simulink model "TestSupervisorFSM_TX"  (R2024b)
settings: Solver=FixedStepDiscrete  StartTime=0.0  StopTime=inf  FixedStep=0.001  RelTol=1e-3  EnableMultiTasking=on
model workspace (MAT data in the model file):
  Command = 1
  State = 0
undefined symbols (not defined in the file): ControlModes
libraries: eeStairGenerator x6
settings Model: DataDictionary=embeddedBoard_common.sldd  Creator=vvasco  LastModifiedBy=mfussi
settings SolverCC: AlgebraicLoopSolver=TrustRegion  AutoInsertRateTranBlk=on
settings DataIOCC: LimitDataPoints=on
settings OptimizationCC: ReuseModelBlockBuffer=off  LifeSpan=inf
settings DebuggingCC: ParameterPrecisionLossMsg=none  UnconnectedInputMsg=warning  UnconnectedOutputMsg=warning  UnconnectedLineMsg=warning  AllowSymbolicDim=off  SFUnexpectedBacktrackingDiag=warning  SFNoUnconditionalDefaultTransitionDiag=warning  SFExecutionAtInitializationDiag=none  ArithmeticOperatorsInVariantConditions=warning
settings ModelReferenceCC: EnableRefExpFcnMdlSchedulingChecks=on
settings SFSimCC: SimUseLocalCustomCode=off  CustomCodeUndefinedFunction=UseInterfaceOnly
settings RTWCC: RTWUseLocalCustomCode=off  GPUComputeCapability=3.5  DLArmComputeVersion=19.05
settings CodeAppCC: StateflowObjectComments=on
settings GRTTargetCC: TargetLangStandard=C89/C90 (ANSI)
settings ConfigComp: CovMetricSettings=dw  CovSaveCumulativeToWorkspaceVar=on  CovSaveSingleToWorkspaceVar=on  CovExternalEMLEnable=off

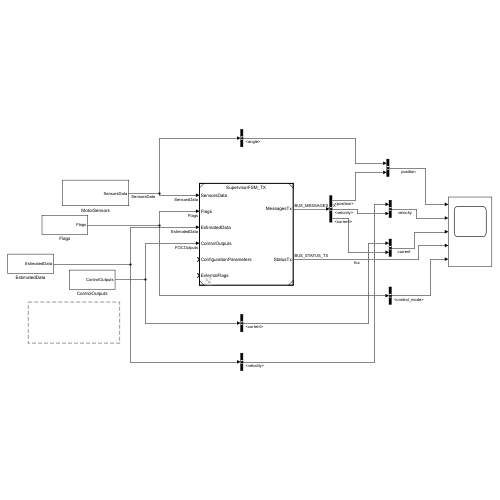
[thumbnail: Simulink's stored preview of the top-level diagram]
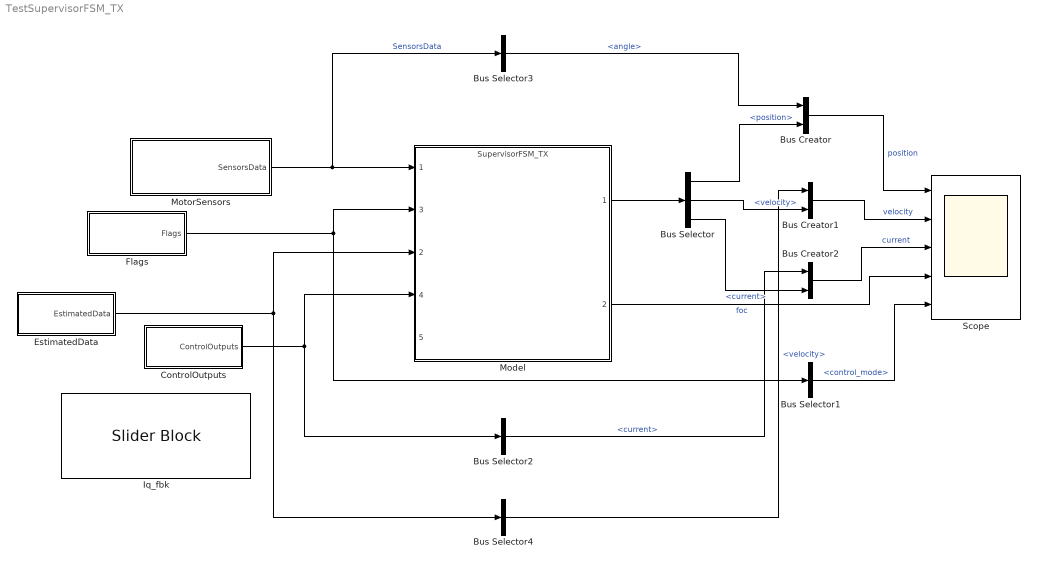
== system TestSupervisorFSM_TX ==
  Bus Creator : BusCreator  Inputs=2
  Bus Creator1 : BusCreator  Inputs=2
  Bus Creator2 : BusCreator  Inputs=2
  Bus Selector : BusSelector  OutputSignals=foc.position,foc.velocity,foc.current
  Bus Selector1 : BusSelector  OutputSignals=control_mode
  Bus Selector2 : BusSelector  OutputSignals=Iq_fbk.current
  Bus Selector3 : BusSelector  OutputSignals=motorsensors.angle
  Bus Selector4 : BusSelector  OutputSignals=jointvelocities.velocity
  ControlOutputs : Subsystem
  EstimatedData : Subsystem
  Flags : Subsystem
  Iq_fbk : SliderBlock  ScaleMax=20
  Model : ModelReference  ModelNameDialog=SupervisorFSM_TX.slx  SimulationMode=Normal  ModelReferenceVersion=9.0
      settings: PortSchema="{\"entries\":[{\"content\":{\"sides\":[{\"content\":{\"connectorIds\":[\"In1\",\"In3\",\"In2\",\"In4\",\"In5\"]},\"type\":\"ConnectorPlacement.EquallySpacedRectSide\",\"uuid\":\"69e4ef43-4003-4440-a894-3828c1af5902\"},{\"content\":{\"connectorIds\":[\"Out1\",\"Out2\"],\"side\":\"RIGHT\"},\"type\":\"ConnectorPlacement.EquallySpacedRectSide\",\"uuid\":\"4c041ecf-670d-4f38-bad4-7d246327a855\"},{\"content\":{\"side\":\"TOP\"},\"type\":\"ConnectorPlacement.EquallySpacedRectSide\",\"uuid\":\"dbbb66c6-d08b-4ab5-92ab-8954eaf6e6e2\"}]},\"type\":\"ConnectorPlacement.EquallySpacedConnector\",\"uuid\":\"4940a0b0-17cd-4df8-8277-6fa028eccbd4\"}],\"packageUris\":[\"http://schema.mathworks.com/mf0/Connector/R2020b\"],\"version\":\"1.0\"}"
  MotorSensors : Subsystem
  Scope : Scope  NumInputPorts=5
  wires:
  Bus Selector/1 -> Bus Creator/2  "<position>"
  Bus Selector3/1 -> Bus Creator/1  "<angle>"
  Bus Creator/1 -> Scope/1  "position"
  Bus Creator1/1 -> Scope/2  "velocity"
  Bus Selector/2 -> Bus Creator1/2  "<velocity>"
  Bus Selector/3 -> Bus Creator2/2  "<current>"
  Bus Creator2/1 -> Scope/3  "current"
  Bus Selector1/1 -> Scope/5  "<control_mode>"
  Model/2 -> Scope/4  "foc"
  Model/1 -> Bus Selector/1
  ControlOutputs/1(ControlOutputs) -> Model/4, Bus Selector2/1
  EstimatedData/1(EstimatedData) -> Model/2, Bus Selector4/1
  MotorSensors/1(SensorsData) -> Bus Selector3/1, Model/1  "SensorsData"
  Bus Selector2/1 -> Bus Creator2/1  "<current>"
  Bus Selector4/1 -> Bus Creator1/1  "<velocity>"
  Flags/1(Flags) -> Bus Selector1/1, Model/3

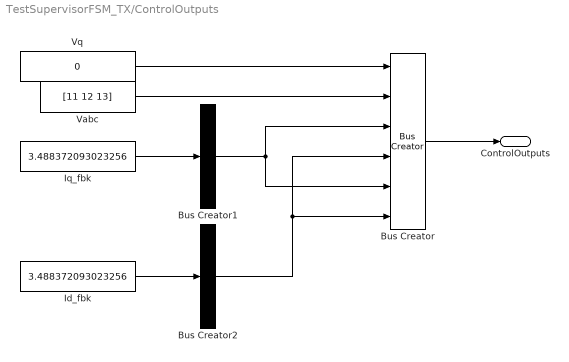
== system TestSupervisorFSM_TX/ControlOutputs ==
  Bus Creator : BusCreator  Inputs=6  OutDataTypeStr=Bus: ControlOutputs
      settings: InheritFromInputs=off
  Bus Creator1 : BusCreator  Inputs=1  OutDataTypeStr=Bus: MotorCurrent
      settings: InheritFromInputs=off
  Bus Creator2 : BusCreator  Inputs=1  OutDataTypeStr=Bus: MotorCurrent
      settings: InheritFromInputs=off
  Id_fbk : Constant  Value=3.488372093023256  OutDataTypeStr=single
  Iq_fbk : Constant  Value=3.488372093023256  OutDataTypeStr=single
  Vabc : Constant  Value=[11 12 13]  OutDataTypeStr=single
  Vq : Constant  Value=0  OutDataTypeStr=single
  ControlOutputs : Outport  OutDataTypeStr=Bus: ControlOutputs
  wires:
  Iq_fbk/1 -> Bus Creator1/1
  Bus Creator/1 -> ControlOutputs/1
  Bus Creator1/1 -> Bus Creator/5, Bus Creator/3
  Vabc/1 -> Bus Creator/2
  Vq/1 -> Bus Creator/1
  Bus Creator2/1 -> Bus Creator/6, Bus Creator/4
  Id_fbk/1 -> Bus Creator2/1

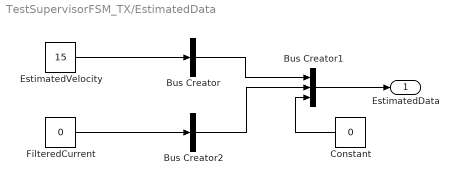
== system TestSupervisorFSM_TX/EstimatedData ==
  Bus Creator : BusCreator  Inputs=1  OutDataTypeStr=Bus: JointVelocities  NonVirtualBus=on
      settings: InheritFromInputs=off
  Bus Creator1 : BusCreator  Inputs=3  OutDataTypeStr=Bus: EstimatedData  NonVirtualBus=on
      settings: InheritFromInputs=off
  Bus Creator2 : BusCreator  Inputs=1  OutDataTypeStr=Bus: MotorCurrent  NonVirtualBus=on
      settings: InheritFromInputs=off
  Constant : Constant  Value=0  OutDataTypeStr=Bus: MotorTemperature
  EstimatedVelocity : Constant  Value=15  OutDataTypeStr=single
  FilteredCurrent : Constant  Value=0  OutDataTypeStr=single
  EstimatedData : Outport
  wires:
  EstimatedVelocity/1 -> Bus Creator/1
  Bus Creator1/1 -> EstimatedData/1
  Bus Creator/1 -> Bus Creator1/1
  FilteredCurrent/1 -> Bus Creator2/1
  Bus Creator2/1 -> Bus Creator1/2
  Constant/1 -> Bus Creator1/3

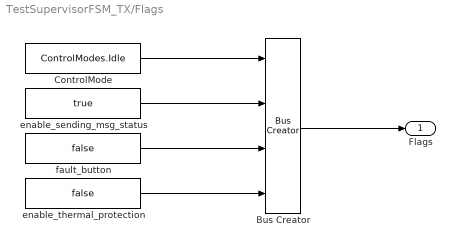
== system TestSupervisorFSM_TX/Flags ==
  Bus Creator : BusCreator  Inputs=4  OutDataTypeStr=Bus: Flags
      settings: InheritFromInputs=off
  ControlMode : Constant  Value=ControlModes.Idle  OutDataTypeStr=Enum: ControlModes
  enable_sending_msg_status : Constant  Value=true  OutDataTypeStr=boolean
  enable_thermal_protection : Constant  Value=false  OutDataTypeStr=boolean
  fault_button : Constant  Value=false  OutDataTypeStr=boolean
  Flags : Outport  OutDataTypeStr=Bus: Flags
  wires:
  ControlMode/1 -> Bus Creator/1
  enable_sending_msg_status/1 -> Bus Creator/2
  Bus Creator/1 -> Flags/1
  fault_button/1 -> Bus Creator/3
  enable_thermal_protection/1 -> Bus Creator/4

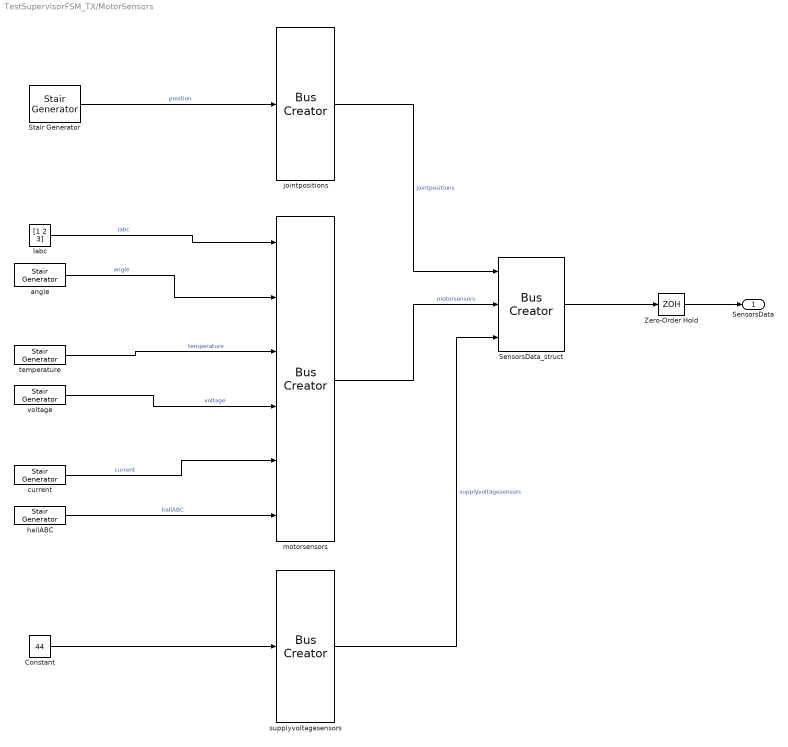
== system TestSupervisorFSM_TX/MotorSensors ==
  Constant : Constant  Value=44  OutDataTypeStr=single
  Iabc : Constant  Value=[1 2 3]  OutDataTypeStr=single
  SensorsData_struct : BusCreator  Inputs=3  OutDataTypeStr=Bus: SensorsData
      settings: InheritFromInputs=off
  Stair Generator : eeStairGenerator/Stair Generator  LabelModeActiveChoice=Discrete  TimeInput=[0.1 0.2 0.3 0.4 0.5 0.6 0.7 0.8 0.9 1 1.1 1.2 1.3 ]  AmplitudeInput=[20 23 26 29 32 35 38 41 39 36 30 25 20]  SampleTime=-1  RepeatPattern=on  OutDataTypeStr=single
  Zero-Order Hold : ZeroOrderHold  SampleTime=0.001
  angle : eeStairGenerator/Stair Generator  LabelModeActiveChoice=Discrete  TimeInput=[0 1 2 3 4 5 6 7 8 9]  AmplitudeInput=[0 1 6 6 6 1 1 1 2 2]  SampleTime=0.1  RepeatPattern=on  OutDataTypeStr=single
  current : eeStairGenerator/Stair Generator  LabelModeActiveChoice=Discrete  TimeInput=[0 0.1 0.2 0.3 0.4 0.5 0.6 0.7 0.8 0.9]  AmplitudeInput=[16 10 15 12 10 16 12 16 18 17]  SampleTime=0.1  RepeatPattern=on  OutDataTypeStr=single
  hallABC : eeStairGenerator/Stair Generator  LabelModeActiveChoice=Discrete  TimeInput=[0 0.1 0.2 0.3 0.4 0.5 0.6 0.7 0.8 0.9]  AmplitudeInput=[6 3 5 2 0 6 6 6 6 6]  SampleTime=-1  RepeatPattern=off  OutDataTypeStr=uint8
  jointpositions : BusCreator  Inputs=position  OutDataTypeStr=Bus: JointPositions
  motorsensors : BusCreator  Inputs=6  OutDataTypeStr=Bus: MotorSensors
  supplyvoltagesensors : BusCreator  Inputs=1  OutDataTypeStr=Bus: SupplyVoltage
  temperature : eeStairGenerator/Stair Generator  LabelModeActiveChoice=Discrete  TimeInput=[0 1 2 3 4 5 6 7 8 9]  AmplitudeInput=[2 2 2 9 9 9 9 9 9 2]  SampleTime=0.1  RepeatPattern=off  OutDataTypeStr=single
  voltage : eeStairGenerator/Stair Generator  LabelModeActiveChoice=Discrete  TimeInput=[0 1 2 3 4 5 6 7 8 9]./10  AmplitudeInput=[2 3 3 3 3 3 2 2 2 2]  SampleTime=0.1  RepeatPattern=on  OutDataTypeStr=single
  SensorsData : Outport  OutDataTypeStr=Bus: SensorsData
  wires:
  motorsensors/1 -> SensorsData_struct/2  "motorsensors"
  voltage/1 -> motorsensors/4  "voltage"
  angle/1 -> motorsensors/2  "angle"
  temperature/1 -> motorsensors/3  "temperature"
  current/1 -> motorsensors/5  "current"
  Iabc/1 -> motorsensors/1  "Iabc"
  hallABC/1 -> motorsensors/6  "hallABC"
  Zero-Order Hold/1 -> SensorsData/1
  Stair Generator/1 -> jointpositions/1  "position"
  SensorsData_struct/1 -> Zero-Order Hold/1
  jointpositions/1 -> SensorsData_struct/1  "jointpositions"
  Constant/1 -> supplyvoltagesensors/1
  supplyvoltagesensors/1 -> SensorsData_struct/3  "supplyvoltagesensors"
